simulink model "MMNNsExample2"  (R2014a)
settings: Solver=ode45  SolverMode=SingleTasking  StartTime=0.0  StopTime=5  RelTol=1e-5
(part 1 of 2)
settings Model: Creator=Administrator  LastModifiedBy=Administrator
settings SolverCC: ZeroCrossControl=DisableAll
settings OptimizationCC: BlockReduction=off  BooleanDataType=off
settings DebuggingCC: SaveWithParameterizedLinksMsg=none  UnderspecifiedInitializationDetection=Classic  SignalResolutionControl=TryResolveAllWithWarning  MaxConsecutiveZCsMsg=none  SolverPrmCheckMsg=none
settings HardwareCC: TargetUnknown=on

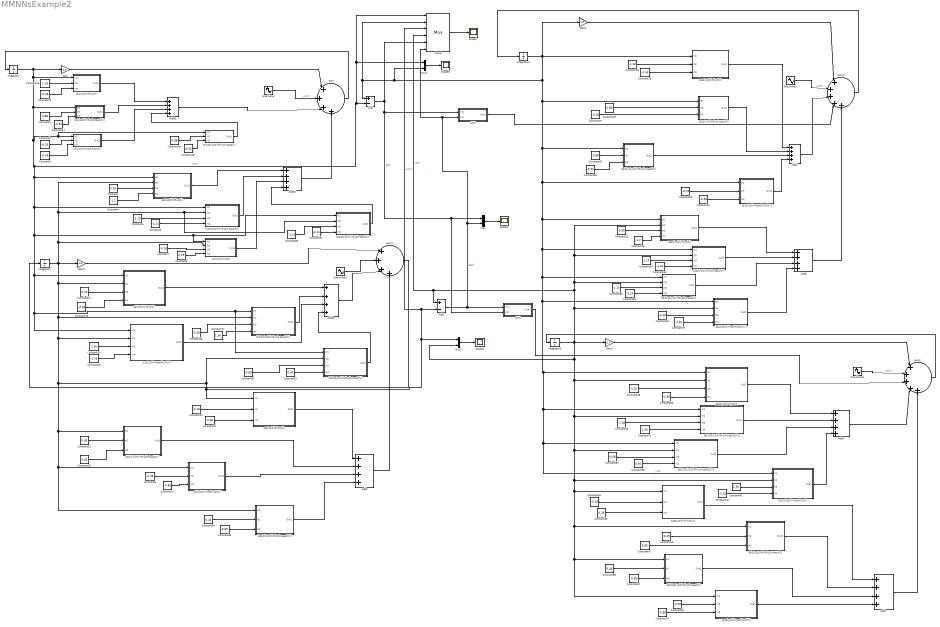
== system MMNNsExample2 ==
  22c21(y2(t))*inst(f(y1(t)) : Subsystem
  2a11(y1(t))*f(y1(t)) : Subsystem
  2a12(y1(t))*f(y2(t)) : Subsystem
  2a21(y2(t))*y1(t)1 : Subsystem
  2a22(x2(t))*f(x2(t))1 : Subsystem
  2b(1)11(y1(t))*f(y1(t-tau2(t))) : Subsystem
  2b(1)21(y2(t))*f(y1(t-tau1(t)))1 : Subsystem
  2b(1)22(y2(t))*f(y2(t-tau(t))1 : Subsystem
  2b(2)12(y1(t))*f(y2(t-tau2(t))) : Subsystem
  2b(2)21(y2(t))*f(y1(t-tau2(t)))1 : Subsystem
  2b(2)22(y2(t))*f(y2(t-tau2(t)) : Subsystem
  2b11(y1(t))*f(y1(t-tau(t))) : Subsystem
  2b12(y1(t))*f(y2(t-tau1(t))) : Subsystem
  2c11(y1(t))*inst(f(y1(t)))1 : Subsystem
  2c12(y1(t))*inst(f(y2(t))))1 : Subsystem
  2c22(y2(t))*inst(f(y2(t))) : Subsystem
  Add : Sum  Inputs=+-
  Add01 : Sum  Inputs=++++
      settings: AttributesFormatString=%<Name>
  Add02 : Sum  Inputs=++++
      settings: AttributesFormatString=%<Name>
  Add03 : Sum  Inputs=++++
      settings: AttributesFormatString=%<Name>
  Add1 : Sum  Inputs=+-
  Add{3..7} (5 alike) : Sum  Inputs=++++
      settings: AttributesFormatString=%<Name>
  Constant : Constant  Value=0.95
  Constant{1,26,48,62} (4 alike) : Constant  Value=0.88
  Constant{10,15,24,39} (4 alike) : Constant  Value=-0.85
      Constant15 settings: AttributesFormatString=%<Name>
      Constant39 settings: AttributesFormatString=%<Name>
  Constant11 : Constant  Value=0.25
      settings: AttributesFormatString=%<Name>
  Constant12 : Constant  Value=1.18
  Constant13 : Constant  Value=-0.45
  Constant{14,27,49,63} (4 alike) : Constant  Value=-0.92
  Constant16 : Constant  Value=-1.68
  Constant17 : Constant  Value=1.56
  Constant18 : Constant  Value=2.56
  Constant19 : Constant  Value=-1.76
  Constant2 : Constant  Value=-0.25
  Constant{7,20,36,44} (4 alike) : Constant  Value=-0.18
  Constant21 : Constant  Value=0.36
  Constant{22,46,54,56} (4 alike) : Constant  Value=0.45
  Constant{23,47,55,57} (4 alike) : Constant  Value=0.85
  Constant25 : Constant  Value=-0.35
  Constant28 : Constant  Value=1.18
  Constant29 : Constant  Value=-0.45
  Constant3 : Constant  Value=-0.56
  Constant30 : Constant  Value=-0.25
  Constant31 : Constant  Value=-0.56
  Constant32 : Constant  Value=0.95
  Constant33 : Constant  Value=-1.2
  Constant34 : Constant  Value=1.15
  Constant35 : Constant  Value=-1.24
  Constant37 : Constant  Value=0.15
  Constant38 : Constant  Value=0.25
      settings: AttributesFormatString=%<Name>
  Constant4 : Constant  Value=-1.2
  Constant40 : Constant  Value=-1.68
  Constant41 : Constant  Value=1.56
  Constant42 : Constant  Value=2.56
  Constant43 : Constant  Value=-1.76
  Constant45 : Constant  Value=0.36
  Constant5 : Constant  Value=1.15
  Constant50 : Constant  Value=-1.15
  Constant51 : Constant  Value=-2.24
  Constant52 : Constant  Value=-0.68
  Constant53 : Constant  Value=0.56
  Constant58 : Constant  Value=0.56
  Constant59 : Constant  Value=-0.68
  Constant6 : Constant  Value=-1.24
  Constant60 : Constant  Value=-1.15
  Constant61 : Constant  Value=-2.24
  Constant8 : Constant  Value=0.15
  Constant9 : Constant  Value=-0.35
  Gain : Gain  Gain=-4.5
  Gain1 : Gain  Gain=-2.5
      settings: AttributesFormatString=|
      | %<Name>
      | %<Gain>
  Gain2 : Gain  Gain=-4.5
      settings: AttributesFormatString=%<Gain>
  Gain3 : Gain  Gain=-2.5
      settings: AttributesFormatString=|
      | %<Name>
      | %<Gain>
  Integrator : Integrator  InitialCondition=0.4
      settings: AttributesFormatString=|
      | %<Name>
      | %<InitialCondition>
  Integrator1 : Integrator  InitialCondition=0.6
      settings: AttributesFormatString=|
      | %<Name>
      | %<InitialCondition>
  Integrator2 : Integrator  InitialCondition=5
      settings: AttributesFormatString=|
      | %<Name>
      | %<InitialCondition>
  Integrator3 : Integrator  InitialCondition=2
      settings: AttributesFormatString=|
      | %<Name>
      | %<InitialCondition>
  Mux : Mux  Inputs=2
  Mux1 : Mux  Inputs=2
  Mux2 : Mux  Inputs=2
  Mux3 : Mux  Inputs=6
  Scope{1..4} (4 alike) : Scope
      Scope1 settings: MaxDataPoints=50000000
      Scope2 settings: AttributesFormatString=%<Name>  YMin=-0.5  MaxDataPoints=50000000
      Scope3 settings: MaxDataPoints=50000000
      Scope4 settings: AttributesFormatString=%<Name>  YMin=-1  SaveName=ScopeData2  MaxDataPoints=50000000
  Sine Wave : Sin  SampleTime=0
      settings: AttributesFormatString=%<Name>
  Sine Wave1 : Sin  Phase=1  SampleTime=0.5*pi
      settings: AttributesFormatString=%<Name>
  Sine Wave2 : Sin  SampleTime=0
  Sine Wave3 : Sin  Phase=pi/2  SampleTime=0
  Sum : Sum  Inputs=|++++
      settings: AttributesFormatString=%<Name>
  Sum1 : Sum  Inputs=|++++
      settings: AttributesFormatString=%<Name>
  Sum2 : Sum  Inputs=|+++++
      settings: AttributesFormatString=%<Name>
  Sum3 : Sum  Inputs=|+++++
      settings: AttributesFormatString=%<Name>
  a11(x1(t))*f(x1(t)) : Subsystem
  a12(x1(t))*f(x2(t)) : Subsystem
  a21(x2(t))*f(x1(t)) : Subsystem
  a22(x2(t))*f(x2(t)) : Subsystem
  b(1)12(x1(t))*f(x2(t-tau1(t))) : Subsystem
  b(1)21(x2(t))*f(x1(t-tau1(t))) : Subsystem
  b(2)11(x1(t))*f(x1(t-tau2t))) : Subsystem
  b(2)12(x1(t))*f(x2(t-tau2(t))) : Subsystem
  b(2)21(x2(t))*f(x1(t-tau2(t))) : Subsystem
  b11(x1(t))*f(x1(t-tau1(t))) : Subsystem
  b22(1)(x2(t))*f(x2(t-tau1(t))) : Subsystem
  b22(2)(x2(t))*f(x2(t-tau2(t))) : Subsystem
  c11(x1(t))*inst(f(x1(t))) : Subsystem
  c12(x1(t))*x2(t) : Subsystem
  c21(x2(t))*inst(f(x1(t))) : Subsystem
  c22(x2(t))*inst(f(x2(t))) : Subsystem
  u1(t) : Subsystem
  u2(t) : Subsystem
  wires:
  a21(x2(t))*f(x1(t))/1(Out1) -> Add03/1
  Integrator/1 -> b(2)11(x1(t))*f(x1(t-tau2t)))/1(In1), c11(x1(t))*inst(f(x1(t)))/1(In1), a12(x1(t))*f(x2(t))/1(In1), b(1)12(x1(t))*f(x2(t-tau1(t)))/1(In1), c21(x2(t))*inst(f(x1(t)))/1(In1), b(2)21(x2(t))*f(x1(t-tau2(t)))/1(In1), b(1)21(x2(t))*f(x1(t-tau1(t)))/1(In1), a21(x2(t))*f(x1(t))/1(In1), b(2)12(x1(t))*f(x2(t-tau2(t)))/1(In1), c12(x1(t))*x2(t)/1(In1), Mux1/1, Mux3/1, Add/2, b11(x1(t))*f(x1(t-tau1(t)))/1(In1), a11(x1(t))*f(x1(t))/1(In1), Gain/1  "x1(t)"
  a12(x1(t))*f(x2(t))/1(Out1) -> Add02/1
  Add02/1 -> Sum/4
  Sine Wave/1 -> Sum/2  "sin(t)"
  Add01/1 -> Sum/3
  Sum/1 -> Integrator/1
  Gain/1 -> Sum/1
  Integrator1/1 -> b(2)12(x1(t))*f(x2(t-tau2(t)))/2(In2), b(1)12(x1(t))*f(x2(t-tau1(t)))/2(In2), a12(x1(t))*f(x2(t))/2(In2), c12(x1(t))*x2(t)/2(In2), Mux2/1, Mux3/3, Add1/2, a22(x2(t))*f(x2(t))/1(In1), b(2)21(x2(t))*f(x1(t-tau2(t)))/2(In2), b22(2)(x2(t))*f(x2(t-tau2(t)))/1(In1), c22(x2(t))*inst(f(x2(t)))/1(In1), b22(1)(x2(t))*f(x2(t-tau1(t)))/1(In1), c21(x2(t))*inst(f(x1(t)))/2(In2), b(1)21(x2(t))*f(x1(t-tau1(t)))/2(In2), a21(x2(t))*f(x1(t))/2(In2), Gain1/1  "x2(t)"
  Gain1/1 -> Sum1/1
  Sine Wave1/1 -> Sum1/2
  Add03/1 -> Sum1/3
  Add3/1 -> Sum1/4
  Gain2/1 -> Sum2/1
  Sum2/1 -> Integrator2/1
  Sine Wave3/1 -> Sum3/2  "cos(t)"
  Gain3/1 -> Sum3/1
  Integrator2/1 -> 2b(1)11(y1(t))*f(y1(t-tau2(t)))/1(In1), 2b(2)12(y1(t))*f(y2(t-tau2(t)))/1(In1), 2a21(y2(t))*y1(t)1/1(In1), 22c21(y2(t))*inst(f(y1(t))/1(In1), 2b(2)21(y2(t))*f(y1(t-tau2(t)))1/1(In1), 2b(1)21(y2(t))*f(y1(t-tau1(t)))1/1(In1), 2c12(y1(t))*inst(f(y2(t))))1/1(In1), 2b12(y1(t))*f(y2(t-tau1(t)))/1(In1), 2a12(y1(t))*f(y2(t))/1(In1), 2c11(y1(t))*inst(f(y1(t)))1/1(In1), 2b11(y1(t))*f(y1(t-tau(t)))/1(In1), Mux1/2, Add/1, Mux3/2, 2a11(y1(t))*f(y1(t))/1(In1), Gain2/1  "y1(t)"
  Sum3/1 -> Integrator3/1
  Add6/1 -> Sum3/4
  Add5/1 -> Sum2/5
  a11(x1(t))*f(x1(t))/1(Out1) -> Add01/1
  b11(x1(t))*f(x1(t-tau1(t)))/1(Out1) -> Add01/2
  c11(x1(t))*inst(f(x1(t)))/1(Out1) -> Add01/3
  b(1)12(x1(t))*f(x2(t-tau1(t)))/1(Out1) -> Add02/2
  c12(x1(t))*x2(t)/1(Out1) -> Add02/3
  2c12(y1(t))*inst(f(y2(t))))1/1(Out1) -> Add5/4
  b(1)21(x2(t))*f(x1(t-tau1(t)))/1(Out1) -> Add03/2
  c21(x2(t))*inst(f(x1(t)))/1(Out1) -> Add03/3
  b22(1)(x2(t))*f(x2(t-tau1(t)))/1(Out1) -> Add3/2
  c22(x2(t))*inst(f(x2(t)))/1(Out1) -> Add3/3
  a22(x2(t))*f(x2(t))/1(Out1) -> Add3/1
  2b(1)22(y2(t))*f(y2(t-tau(t))1/1(Out1) -> Add7/2
  Sine Wave2/1 -> Sum2/2  "sin(t)"
  Add4/1 -> Sum2/3
  Add/1 -> u1(t)/1(In1), u2(t)/2(In2), Mux/1, Mux3/5  "e1(t)"
  Add1/1 -> u2(t)/1(In1), Mux/2, u1(t)/2(In2), Mux3/6  "e2(t)"
  Sum1/1 -> Integrator1/1
  Mux/1 -> Scope2/1
  Add7/1 -> Sum3/5
  Constant12/1 -> a11(x1(t))*f(x1(t))/2(In2)
  Constant13/1 -> a11(x1(t))*f(x1(t))/3(In3)
  Constant1/1 -> b11(x1(t))*f(x1(t-tau1(t)))/2(In2)
  Constant14/1 -> b11(x1(t))*f(x1(t-tau1(t)))/3(In3)
  Constant2/1 -> c11(x1(t))*inst(f(x1(t)))/2(In2)
  Constant3/1 -> c11(x1(t))*inst(f(x1(t)))/3(In3)
  Constant/1 -> a12(x1(t))*f(x2(t))/3(In3)
  Constant4/1 -> a12(x1(t))*f(x2(t))/4(In4)
  Constant5/1 -> b(1)12(x1(t))*f(x2(t-tau1(t)))/3(In3)
  Constant6/1 -> b(1)12(x1(t))*f(x2(t-tau1(t)))/4(In4)
  Constant7/1 -> c12(x1(t))*x2(t)/3(In3)
  Constant8/1 -> c12(x1(t))*x2(t)/4(In4)
  Constant9/1 -> c22(x2(t))*inst(f(x2(t)))/2(In2)
  Constant10/1 -> c22(x2(t))*inst(f(x2(t)))/3(In3)
  Constant15/1 -> a21(x2(t))*f(x1(t))/4(In4)
  Constant11/1 -> a21(x2(t))*f(x1(t))/3(In3)
  Constant16/1 -> b(1)21(x2(t))*f(x1(t-tau1(t)))/3(In3)
  Constant17/1 -> b(1)21(x2(t))*f(x1(t-tau1(t)))/4(In4)
  Constant18/1 -> c21(x2(t))*inst(f(x1(t)))/3(In3)
  Constant19/1 -> c21(x2(t))*inst(f(x1(t)))/4(In4)
  Constant20/1 -> a22(x2(t))*f(x2(t))/2(In2)
  Constant21/1 -> a22(x2(t))*f(x2(t))/3(In3)
  Constant22/1 -> b22(1)(x2(t))*f(x2(t-tau1(t)))/2(In2)
  Constant23/1 -> b22(1)(x2(t))*f(x2(t-tau1(t)))/3(In3)
  Constant25/1 -> 2c22(y2(t))*inst(f(y2(t)))/2(In2)
  Constant24/1 -> 2c22(y2(t))*inst(f(y2(t)))/3(In3)
  2c22(y2(t))*inst(f(y2(t)))/1(Out1) -> Add7/4
  Constant28/1 -> 2a11(y1(t))*f(y1(t))/2(In2)
  Constant29/1 -> 2a11(y1(t))*f(y1(t))/3(In3)
  Constant26/1 -> 2b11(y1(t))*f(y1(t-tau(t)))/2(In2)
  Constant27/1 -> 2b11(y1(t))*f(y1(t-tau(t)))/3(In3)
  Constant31/1 -> 2c11(y1(t))*inst(f(y1(t)))1/3(In3)
  Constant30/1 -> 2c11(y1(t))*inst(f(y1(t)))1/2(In2)
  2a11(y1(t))*f(y1(t))/1(Out1) -> Add4/1
  2b11(y1(t))*f(y1(t-tau(t)))/1(Out1) -> Add4/2
  2c11(y1(t))*inst(f(y1(t)))1/1(Out1) -> Add4/4
  Constant32/1 -> 2a12(y1(t))*f(y2(t))/3(In3)
  Constant33/1 -> 2a12(y1(t))*f(y2(t))/4(In4)
  2a12(y1(t))*f(y2(t))/1(Out1) -> Add5/1
  Constant34/1 -> 2b12(y1(t))*f(y2(t-tau1(t)))/3(In3)
  Constant35/1 -> 2b12(y1(t))*f(y2(t-tau1(t)))/4(In4)
  2b12(y1(t))*f(y2(t-tau1(t)))/1(Out1) -> Add5/2
  Constant36/1 -> 2c12(y1(t))*inst(f(y2(t))))1/3(In3)
  Constant37/1 -> 2c12(y1(t))*inst(f(y2(t))))1/4(In4)
  Constant38/1 -> 2a21(y2(t))*y1(t)1/3(In3)
  Constant39/1 -> 2a21(y2(t))*y1(t)1/4(In4)
  Constant40/1 -> 2b(1)21(y2(t))*f(y1(t-tau1(t)))1/3(In3)
  Constant41/1 -> 2b(1)21(y2(t))*f(y1(t-tau1(t)))1/4(In4)
  2b(1)21(y2(t))*f(y1(t-tau1(t)))1/1(Out1) -> Add6/2
  Constant43/1 -> 22c21(y2(t))*inst(f(y1(t))/4(In4)
  Constant42/1 -> 22c21(y2(t))*inst(f(y1(t))/3(In3)
  22c21(y2(t))*inst(f(y1(t))/1(Out1) -> Add6/4
  2a21(y2(t))*y1(t)1/1(Out1) -> Add6/1
  Constant44/1 -> 2a22(x2(t))*f(x2(t))1/2(In2)
  Constant45/1 -> 2a22(x2(t))*f(x2(t))1/3(In3)
  2a22(x2(t))*f(x2(t))1/1(Out1) -> Add7/1
  Constant46/1 -> 2b(1)22(y2(t))*f(y2(t-tau(t))1/2(In2)
  Constant47/1 -> 2b(1)22(y2(t))*f(y2(t-tau(t))1/3(In3)
  Mux1/1 -> Scope3/1
  Mux2/1 -> Scope4/1
  u1(t)/1(Out1) -> Sum2/4
  Constant48/1 -> b(2)11(x1(t))*f(x1(t-tau2t)))/2(In2)
  Constant49/1 -> b(2)11(x1(t))*f(x1(t-tau2t)))/3(In3)
  b(2)11(x1(t))*f(x1(t-tau2t)))/1(Out1) -> Add01/4
  Constant51/1 -> b(2)12(x1(t))*f(x2(t-tau2(t)))/4(In4)
  Constant50/1 -> b(2)12(x1(t))*f(x2(t-tau2(t)))/3(In3)
  b(2)12(x1(t))*f(x2(t-tau2(t)))/1(Out1) -> Add02/4
  Constant53/1 -> b(2)21(x2(t))*f(x1(t-tau2(t)))/4(In4)
  Constant52/1 -> b(2)21(x2(t))*f(x1(t-tau2(t)))/3(In3)
  b(2)21(x2(t))*f(x1(t-tau2(t)))/1(Out1) -> Add03/4
  Constant55/1 -> b22(2)(x2(t))*f(x2(t-tau2(t)))/3(In3)
  Constant54/1 -> b22(2)(x2(t))*f(x2(t-tau2(t)))/2(In2)
  b22(2)(x2(t))*f(x2(t-tau2(t)))/1(Out1) -> Add3/4
  Constant57/1 -> 2b(2)22(y2(t))*f(y2(t-tau2(t))/3(In3)
  Integrator3/1 -> 2a12(y1(t))*f(y2(t))/2(In2), 2b12(y1(t))*f(y2(t-tau1(t)))/2(In2), 2b(2)12(y1(t))*f(y2(t-tau2(t)))/2(In2), Mux3/4, Add1/1, 2c12(y1(t))*inst(f(y2(t))))1/2(In2), Gain3/1, Mux2/2, 2a21(y2(t))*y1(t)1/2(In2), 2b(1)21(y2(t))*f(y1(t-tau1(t)))1/2(In2), 2b(2)21(y2(t))*f(y1(t-tau2(t)))1/2(In2), 2a22(x2(t))*f(x2(t))1/1(In1), 2c22(y2(t))*inst(f(y2(t)))/1(In1), 2b(2)22(y2(t))*f(y2(t-tau2(t))/1(In1), 2b(1)22(y2(t))*f(y2(t-tau(t))1/1(In1), 22c21(y2(t))*inst(f(y1(t))/2(In2)  "y2(t)"
  Constant56/1 -> 2b(2)22(y2(t))*f(y2(t-tau2(t))/2(In2)
  2b(2)22(y2(t))*f(y2(t-tau2(t))/1(Out1) -> Add7/3
  Constant59/1 -> 2b(2)21(y2(t))*f(y1(t-tau2(t)))1/3(In3)
  Constant58/1 -> 2b(2)21(y2(t))*f(y1(t-tau2(t)))1/4(In4)
  2b(2)21(y2(t))*f(y1(t-tau2(t)))1/1(Out1) -> Add6/3
  Constant61/1 -> 2b(2)12(y1(t))*f(y2(t-tau2(t)))/4(In4)
  Constant60/1 -> 2b(2)12(y1(t))*f(y2(t-tau2(t)))/3(In3)
  2b(2)12(y1(t))*f(y2(t-tau2(t)))/1(Out1) -> Add5/3
  Constant63/1 -> 2b(1)11(y1(t))*f(y1(t-tau2(t)))/3(In3)
  Constant62/1 -> 2b(1)11(y1(t))*f(y1(t-tau2(t)))/2(In2)
  2b(1)11(y1(t))*f(y1(t-tau2(t)))/1(Out1) -> Add4/3
  u2(t)/1(Out1) -> Sum3/3
  Mux3/1 -> Scope1/1

== system MMNNsExample2/22c21(y2(t))*inst(f(y1(t)) ==
  In1 : Inport
      settings: AttributesFormatString=%<Name>
  In2 : Inport  Port=2
      settings: AttributesFormatString=%<Name>
  In3 : Inport  Port=3
      settings: AttributesFormatString=%<Name>
  In4 : Inport  Port=4
      settings: AttributesFormatString=%<Name>
  Abs : Abs
  Subsystem : Subsystem
  Switch : Switch  Criteria=u2 > Threshold  Threshold=1
  Out1 : Outport
  wires:
  In1/1 -> Subsystem/2(In2)  "x1(t)"
  Subsystem/1(Out1) -> Out1/1
  Abs/1 -> Switch/2
  In3/1 -> Switch/1
  In4/1 -> Switch/3
  Switch/1 -> Subsystem/1(In1)
  In2/1 -> Abs/1  "x2(t)"

== system MMNNsExample2/2a11(y1(t))*f(y1(t)) ==
  In1 : Inport
  In2 : Inport  Port=2
  In3 : Inport  Port=3
  Abs3 : Abs
  Switch4 : Switch  Criteria=u2 > Threshold  Threshold=1
  a11(x1(t))*x1(t) : Subsystem
  Out1 : Outport
  wires:
  a11(x1(t))*x1(t)/1(Out1) -> Out1/1
  Abs3/1 -> Switch4/2
  In2/1 -> Switch4/1
  In3/1 -> Switch4/3
  In1/1 -> a11(x1(t))*x1(t)/2(In2), Abs3/1  "x1(t)"
  Switch4/1 -> a11(x1(t))*x1(t)/1(ln1)

== system MMNNsExample2/2a12(y1(t))*f(y2(t)) ==
  In1 : Inport
      settings: AttributesFormatString=%<Name>
  In2 : Inport  Port=2
      settings: AttributesFormatString=%<Name>
  In3 : Inport  Port=3
      settings: AttributesFormatString=%<Name>
  In4 : Inport  Port=4
      settings: AttributesFormatString=%<Name>
  Abs : Abs
  Subsystem : Subsystem
  Switch : Switch  Criteria=u2 > Threshold  Threshold=1
  Out1 : Outport
  wires:
  In1/1 -> Abs/1  "x1(t)"
  Switch/1 -> Subsystem/1(In1)
  In2/1 -> Subsystem/2(In2)  "x2(t)"
  Subsystem/1(Out1) -> Out1/1
  Abs/1 -> Switch/2
  In3/1 -> Switch/1
  In4/1 -> Switch/3

== system MMNNsExample2/2a21(y2(t))*y1(t)1 ==
  In1 : Inport
      settings: AttributesFormatString=%<Name>
  In2 : Inport  Port=2
      settings: AttributesFormatString=%<Name>
  In3 : Inport  Port=3
      settings: AttributesFormatString=%<Name>
  In4 : Inport  Port=4
      settings: AttributesFormatString=%<Name>
  Abs : Abs
      settings: AttributesFormatString=%<Name>
  Product : Product
      settings: AttributesFormatString=%<Name>
  Switch : Switch  Criteria=u2 > Threshold  Threshold=1
  f1(x1(t))=(|x+1|-|x-1|)/2 : Subsystem
  Out1 : Outport
      settings: AttributesFormatString=%<Name>
  wires:
  Product/1 -> Out1/1
  In2/1 -> Abs/1  "x2(t)"
  f1(x1(t))=(|x+1|-|x-1|)/2/1(Out1) -> Product/2
  In1/1 -> f1(x1(t))=(|x+1|-|x-1|)/2/1(In1)  "x1(t)"
  In4/1 -> Switch/1
  Switch/1 -> Product/1
  Abs/1 -> Switch/2
  In3/1 -> Switch/3

== system MMNNsExample2/2a22(x2(t))*f(x2(t))1 ==
  In1 : Inport
  In2 : Inport  Port=2
  In3 : Inport  Port=3
  Abs3 : Abs
  Switch4 : Switch  Criteria=u2 > Threshold  Threshold=1
  a22(x2(t))*x2(t) : Subsystem
  Out1 : Outport
  wires:
  a22(x2(t))*x2(t)/1(Out1) -> Out1/1
  In1/1 -> a22(x2(t))*x2(t)/2(In2), Abs3/1  "x2(t)"
  Switch4/1 -> a22(x2(t))*x2(t)/1(ln1)
  Abs3/1 -> Switch4/2
  In3/1 -> Switch4/3
  In2/1 -> Switch4/1

== system MMNNsExample2/2b(1)11(y1(t))*f(y1(t-tau2(t))) ==
  In1 : Inport
  In2 : Inport  Port=2
  In3 : Inport  Port=3
  Abs1 : Abs
  Switch1 : Switch  Criteria=u2 > Threshold  Threshold=1
  x1(t)*b11(x1(t)) : Subsystem
  Out1 : Outport
  wires:
  In1/1 -> x1(t)*b11(x1(t))/2(In2), Abs1/1  "x1(t)"
  x1(t)*b11(x1(t))/1(Out1) -> Out1/1
  Switch1/1 -> x1(t)*b11(x1(t))/1(In1)  "b11(x1(t))"
  In3/1 -> Switch1/1
  In2/1 -> Switch1/3
  Abs1/1 -> Switch1/2

== system MMNNsExample2/2b(1)21(y2(t))*f(y1(t-tau1(t)))1 ==
  In1 : Inport
      settings: AttributesFormatString=%<Name>
  In2 : Inport  Port=2
      settings: AttributesFormatString=%<Name>
  In3 : Inport  Port=3
      settings: AttributesFormatString=%<Name>
  In4 : Inport  Port=4
      settings: AttributesFormatString=%<Name>
  Abs : Abs
  Subsystem : Subsystem
  Switch : Switch  Criteria=u2 > Threshold  Threshold=1
      settings: AttributesFormatString=%<Name>
  Out1 : Outport
  wires:
  In1/1 -> Subsystem/2(In2)  "x1(t)"
  In2/1 -> Abs/1  "x2(t)"
  Subsystem/1(Out1) -> Out1/1
  In4/1 -> Switch/3
  In3/1 -> Switch/1
  Abs/1 -> Switch/2
  Switch/1 -> Subsystem/1(In1)  "b21"

== system MMNNsExample2/2b(1)22(y2(t))*f(y2(t-tau(t))1 ==
  In1 : Inport
  In2 : Inport  Port=2
  In3 : Inport  Port=3
  Abs1 : Abs
  Switch1 : Switch  Criteria=u2 > Threshold  Threshold=1
  x2(t)*b22(x2(t)) : Subsystem
  Out1 : Outport
  wires:
  In1/1 -> Abs1/1, x2(t)*b22(x2(t))/2(In2)  "x2(t)"
  x2(t)*b22(x2(t))/1(Out1) -> Out1/1
  In2/1 -> Switch1/1
  Abs1/1 -> Switch1/2
  In3/1 -> Switch1/3
  Switch1/1 -> x2(t)*b22(x2(t))/1(In1)

== system MMNNsExample2/2b(2)12(y1(t))*f(y2(t-tau2(t))) ==
  In1 : Inport
  In2 : Inport  Port=2
  In3 : Inport  Port=3
  In4 : Inport  Port=4
  Abs : Abs
  Subsystem : Subsystem
  Switch : Switch  Criteria=u2 > Threshold  Threshold=1
  Out1 : Outport
      settings: AttributesFormatString=%<Name>
  wires:
  Subsystem/1(Out1) -> Out1/1
  In3/1 -> Switch/1
  In4/1 -> Switch/3
  Switch/1 -> Subsystem/1(In1)  "b12"
  Abs/1 -> Switch/2
  In1/1 -> Abs/1  "x1(t)"
  In2/1 -> Subsystem/2(In2)

== system MMNNsExample2/2b(2)21(y2(t))*f(y1(t-tau2(t)))1 ==
  In1 : Inport
      settings: AttributesFormatString=%<Name>
  In2 : Inport  Port=2
      settings: AttributesFormatString=%<Name>
  In3 : Inport  Port=3
      settings: AttributesFormatString=%<Name>
  In4 : Inport  Port=4
      settings: AttributesFormatString=%<Name>
  Abs : Abs
  Subsystem : Subsystem
  Switch : Switch  Criteria=u2 > Threshold  Threshold=1
      settings: AttributesFormatString=%<Name>
  Out1 : Outport
  wires:
  In1/1 -> Subsystem/2(In2)  "x1(t)"
  In2/1 -> Abs/1  "x2(t)"
  Subsystem/1(Out1) -> Out1/1
  In4/1 -> Switch/3
  In3/1 -> Switch/1
  Abs/1 -> Switch/2
  Switch/1 -> Subsystem/1(In1)  "b21"

== system MMNNsExample2/2b(2)22(y2(t))*f(y2(t-tau2(t)) ==
  In1 : Inport
  In2 : Inport  Port=2
  In3 : Inport  Port=3
  Abs1 : Abs
  Switch1 : Switch  Criteria=u2 > Threshold  Threshold=1
  x2(t)*b22(x2(t)) : Subsystem
  Out1 : Outport
  wires:
  In1/1 -> Abs1/1, x2(t)*b22(x2(t))/2(In2)  "x2(t)"
  x2(t)*b22(x2(t))/1(Out1) -> Out1/1
  In2/1 -> Switch1/1
  Abs1/1 -> Switch1/2
  In3/1 -> Switch1/3
  Switch1/1 -> x2(t)*b22(x2(t))/1(In1)

== system MMNNsExample2/2b11(y1(t))*f(y1(t-tau(t))) ==
  In1 : Inport
  In2 : Inport  Port=2
  In3 : Inport  Port=3
  Abs1 : Abs
  Switch1 : Switch  Criteria=u2 > Threshold  Threshold=1
  x1(t)*b11(x1(t)) : Subsystem
  Out1 : Outport
  wires:
  In1/1 -> x1(t)*b11(x1(t))/2(In2), Abs1/1  "x1(t)"
  x1(t)*b11(x1(t))/1(Out1) -> Out1/1
  Switch1/1 -> x1(t)*b11(x1(t))/1(In1)  "b11(x1(t))"
  In3/1 -> Switch1/1
  In2/1 -> Switch1/3
  Abs1/1 -> Switch1/2

== system MMNNsExample2/2b12(y1(t))*f(y2(t-tau1(t))) ==
  In1 : Inport
  In2 : Inport  Port=2
  In3 : Inport  Port=3
  In4 : Inport  Port=4
  Abs : Abs
  Subsystem : Subsystem
  Switch : Switch  Criteria=u2 > Threshold  Threshold=1
  Out1 : Outport
      settings: AttributesFormatString=%<Name>
  wires:
  Subsystem/1(Out1) -> Out1/1
  In3/1 -> Switch/1
  In4/1 -> Switch/3
  Switch/1 -> Subsystem/1(In1)  "b12"
  Abs/1 -> Switch/2
  In1/1 -> Abs/1  "x1(t)"
  In2/1 -> Subsystem/2(In2)

== system MMNNsExample2/2c11(y1(t))*inst(f(y1(t)))1 ==
  In1 : Inport
      settings: AttributesFormatString=%<Name>
  In2 : Inport  Port=2
      settings: AttributesFormatString=%<Name>
  In3 : Inport  Port=3
      settings: AttributesFormatString=%<Name>
  Abs3 : Abs
  Switch4 : Switch  Criteria=u2 > Threshold  Threshold=1
  c11*inst(f1(x1(t))) : Subsystem
  Out1 : Outport
  wires:
  c11*inst(f1(x1(t)))/1(Out1) -> Out1/1
  In1/1 -> Abs3/1, c11*inst(f1(x1(t)))/2(In2)  "x1(t)"
  Abs3/1 -> Switch4/2
  Switch4/1 -> c11*inst(f1(x1(t)))/1(In1)  "c11"
  In2/1 -> Switch4/1
  In3/1 -> Switch4/3

== system MMNNsExample2/2c12(y1(t))*inst(f(y2(t))))1 ==
  In1 : Inport
      settings: AttributesFormatString=%<Name>
  In2 : Inport  Port=2
      settings: AttributesFormatString=%<Name>
  In3 : Inport  Port=3
      settings: AttributesFormatString=%<Name>
  In4 : Inport  Port=4
      settings: AttributesFormatString=%<Name>
  Abs : Abs
  Subsystem : Subsystem
  Switch : Switch  Criteria=u2 > Threshold  Threshold=1
  Out1 : Outport
  wires:
  In1/1 -> Abs/1  "x1(t)"
  In2/1 -> Subsystem/2(In2)  "x2(t)"
  Subsystem/1(Out1) -> Out1/1
  Switch/1 -> Subsystem/1(In1)
  Abs/1 -> Switch/2
  In3/1 -> Switch/1
  In4/1 -> Switch/3

== system MMNNsExample2/2c22(y2(t))*inst(f(y2(t))) ==
  In1 : Inport
  In2 : Inport  Port=2
  In3 : Inport  Port=3
  Abs3 : Abs
  Switch4 : Switch  Criteria=u2 > Threshold  Threshold=1
  c22*inst(f2(x2(t))) : Subsystem
  Out1 : Outport
  wires:
  c22*inst(f2(x2(t)))/1(Out1) -> Out1/1
  In1/1 -> c22*inst(f2(x2(t)))/2(In2), Abs3/1  "x2(t)"
  Switch4/1 -> c22*inst(f2(x2(t)))/1(In1)  "c11"
  In2/1 -> Switch4/1
  Abs3/1 -> Switch4/2
  In3/1 -> Switch4/3

== system MMNNsExample2/a11(x1(t))*f(x1(t)) ==
  In1 : Inport
  In2 : Inport  Port=2
  In3 : Inport  Port=3
  Abs3 : Abs
  Switch4 : Switch  Criteria=u2 > Threshold  Threshold=1
  a11(x1(t))*x1(t) : Subsystem
  Out1 : Outport
  wires:
  a11(x1(t))*x1(t)/1(Out1) -> Out1/1
  Abs3/1 -> Switch4/2
  In2/1 -> Switch4/1
  In3/1 -> Switch4/3
  In1/1 -> a11(x1(t))*x1(t)/2(In2), Abs3/1  "x1(t)"
  Switch4/1 -> a11(x1(t))*x1(t)/1(ln1)

== system MMNNsExample2/a12(x1(t))*f(x2(t)) ==
  In1 : Inport
      settings: AttributesFormatString=%<Name>
  In2 : Inport  Port=2
      settings: AttributesFormatString=%<Name>
  In3 : Inport  Port=3
      settings: AttributesFormatString=%<Name>
  In4 : Inport  Port=4
      settings: AttributesFormatString=%<Name>
  Abs : Abs
  Subsystem : Subsystem
  Switch : Switch  Criteria=u2 > Threshold  Threshold=1
  Out1 : Outport
  wires:
  In1/1 -> Abs/1  "x1(t)"
  Switch/1 -> Subsystem/1(In1)
  In2/1 -> Subsystem/2(In2)  "x2(t)"
  Subsystem/1(Out1) -> Out1/1
  Abs/1 -> Switch/2
  In3/1 -> Switch/1
  In4/1 -> Switch/3

== system MMNNsExample2/a21(x2(t))*f(x1(t)) ==
  In1 : Inport
      settings: AttributesFormatString=%<Name>
  In2 : Inport  Port=2
      settings: AttributesFormatString=%<Name>
  In3 : Inport  Port=3
      settings: AttributesFormatString=%<Name>
  In4 : Inport  Port=4
      settings: AttributesFormatString=%<Name>
  Abs : Abs
      settings: AttributesFormatString=%<Name>
  Product : Product
      settings: AttributesFormatString=%<Name>
  Switch : Switch  Criteria=u2 > Threshold  Threshold=1
  f1(x1(t))=(|x+1|-|x-1|)/2 : Subsystem
  Out1 : Outport
      settings: AttributesFormatString=%<Name>
  wires:
  Product/1 -> Out1/1
  In2/1 -> Abs/1  "x2(t)"
  f1(x1(t))=(|x+1|-|x-1|)/2/1(Out1) -> Product/2
  In1/1 -> f1(x1(t))=(|x+1|-|x-1|)/2/1(In1)  "x1(t)"
  In4/1 -> Switch/1
  Switch/1 -> Product/1
  Abs/1 -> Switch/2
  In3/1 -> Switch/3

== system MMNNsExample2/a22(x2(t))*f(x2(t)) ==
  In1 : Inport
  In2 : Inport  Port=2
  In3 : Inport  Port=3
  Abs3 : Abs
  Switch4 : Switch  Criteria=u2 > Threshold  Threshold=1
  a22(x2(t))*x2(t) : Subsystem
  Out1 : Outport
  wires:
  a22(x2(t))*x2(t)/1(Out1) -> Out1/1
  In1/1 -> a22(x2(t))*x2(t)/2(In2), Abs3/1  "x2(t)"
  Switch4/1 -> a22(x2(t))*x2(t)/1(ln1)
  Abs3/1 -> Switch4/2
  In3/1 -> Switch4/3
  In2/1 -> Switch4/1

== system MMNNsExample2/b(1)12(x1(t))*f(x2(t-tau1(t))) ==
  In1 : Inport
  In2 : Inport  Port=2
  In3 : Inport  Port=3
  In4 : Inport  Port=4
  Abs : Abs
  Subsystem : Subsystem
  Switch : Switch  Criteria=u2 > Threshold  Threshold=1
  Out1 : Outport
      settings: AttributesFormatString=%<Name>
  wires:
  Subsystem/1(Out1) -> Out1/1
  In3/1 -> Switch/1
  In4/1 -> Switch/3
  Switch/1 -> Subsystem/1(In1)  "b12"
  Abs/1 -> Switch/2
  In1/1 -> Abs/1  "x1(t)"
  In2/1 -> Subsystem/2(In2)

== system MMNNsExample2/b(1)21(x2(t))*f(x1(t-tau1(t))) ==
  In1 : Inport
      settings: AttributesFormatString=%<Name>
  In2 : Inport  Port=2
      settings: AttributesFormatString=%<Name>
  In3 : Inport  Port=3
      settings: AttributesFormatString=%<Name>
  In4 : Inport  Port=4
      settings: AttributesFormatString=%<Name>
  Abs : Abs
  Subsystem : Subsystem
  Switch : Switch  Criteria=u2 > Threshold  Threshold=1
      settings: AttributesFormatString=%<Name>
  Out1 : Outport
  wires:
  In1/1 -> Subsystem/2(In2)  "x1(t)"
  In2/1 -> Abs/1  "x2(t)"
  Subsystem/1(Out1) -> Out1/1
  In4/1 -> Switch/3
  In3/1 -> Switch/1
  Abs/1 -> Switch/2
  Switch/1 -> Subsystem/1(In1)  "b21"

== system MMNNsExample2/b(2)11(x1(t))*f(x1(t-tau2t))) ==
  In1 : Inport
  In2 : Inport  Port=2
  In3 : Inport  Port=3
  Abs1 : Abs
  Switch1 : Switch  Criteria=u2 > Threshold  Threshold=1
  x1(t)*b11(x1(t)) : Subsystem
  Out1 : Outport
  wires:
  In1/1 -> x1(t)*b11(x1(t))/2(In2), Abs1/1  "x1(t)"
  x1(t)*b11(x1(t))/1(Out1) -> Out1/1
  Switch1/1 -> x1(t)*b11(x1(t))/1(In1)  "b11(x1(t))"
  In3/1 -> Switch1/1
  In2/1 -> Switch1/3
  Abs1/1 -> Switch1/2

== system MMNNsExample2/b(2)12(x1(t))*f(x2(t-tau2(t))) ==
  In1 : Inport
  In2 : Inport  Port=2
  In3 : Inport  Port=3
  In4 : Inport  Port=4
  Abs : Abs
  Subsystem : Subsystem
  Switch : Switch  Criteria=u2 > Threshold  Threshold=1
  Out1 : Outport
      settings: AttributesFormatString=%<Name>
  wires:
  Subsystem/1(Out1) -> Out1/1
  In3/1 -> Switch/1
  In4/1 -> Switch/3
  Switch/1 -> Subsystem/1(In1)  "b12"
  Abs/1 -> Switch/2
  In1/1 -> Abs/1  "x1(t)"
  In2/1 -> Subsystem/2(In2)

== system MMNNsExample2/b(2)21(x2(t))*f(x1(t-tau2(t))) ==
  In1 : Inport
      settings: AttributesFormatString=%<Name>
  In2 : Inport  Port=2
      settings: AttributesFormatString=%<Name>
  In3 : Inport  Port=3
      settings: AttributesFormatString=%<Name>
  In4 : Inport  Port=4
      settings: AttributesFormatString=%<Name>
  Abs : Abs
  Subsystem : Subsystem
  Switch : Switch  Criteria=u2 > Threshold  Threshold=1
      settings: AttributesFormatString=%<Name>
  Out1 : Outport
  wires:
  In1/1 -> Subsystem/2(In2)  "x1(t)"
  In2/1 -> Abs/1  "x2(t)"
  Subsystem/1(Out1) -> Out1/1
  In4/1 -> Switch/3
  In3/1 -> Switch/1
  Abs/1 -> Switch/2
  Switch/1 -> Subsystem/1(In1)  "b21"

== system MMNNsExample2/b11(x1(t))*f(x1(t-tau1(t))) ==
  In1 : Inport
  In2 : Inport  Port=2
  In3 : Inport  Port=3
  Abs1 : Abs
  Switch1 : Switch  Criteria=u2 > Threshold  Threshold=1
  x1(t)*b11(x1(t)) : Subsystem
  Out1 : Outport
  wires:
  In1/1 -> x1(t)*b11(x1(t))/2(In2), Abs1/1  "x1(t)"
  x1(t)*b11(x1(t))/1(Out1) -> Out1/1
  Switch1/1 -> x1(t)*b11(x1(t))/1(In1)  "b11(x1(t))"
  In3/1 -> Switch1/1
  In2/1 -> Switch1/3
  Abs1/1 -> Switch1/2

== system MMNNsExample2/b22(1)(x2(t))*f(x2(t-tau1(t))) ==
  In1 : Inport
  In2 : Inport  Port=2
  In3 : Inport  Port=3
  Abs1 : Abs
  Switch1 : Switch  Criteria=u2 > Threshold  Threshold=1
  x2(t)*b22(x2(t)) : Subsystem
  Out1 : Outport
  wires:
  In1/1 -> Abs1/1, x2(t)*b22(x2(t))/2(In2)  "x2(t)"
  x2(t)*b22(x2(t))/1(Out1) -> Out1/1
  In2/1 -> Switch1/1
  Abs1/1 -> Switch1/2
  In3/1 -> Switch1/3
  Switch1/1 -> x2(t)*b22(x2(t))/1(In1)

== system MMNNsExample2/b22(2)(x2(t))*f(x2(t-tau2(t))) ==
  In1 : Inport
  In2 : Inport  Port=2
  In3 : Inport  Port=3
  Abs1 : Abs
  Switch1 : Switch  Criteria=u2 > Threshold  Threshold=1
  x2(t)*b22(x2(t)) : Subsystem
  Out1 : Outport
  wires:
  In1/1 -> Abs1/1, x2(t)*b22(x2(t))/2(In2)  "x2(t)"
  x2(t)*b22(x2(t))/1(Out1) -> Out1/1
  In2/1 -> Switch1/1
  Abs1/1 -> Switch1/2
  In3/1 -> Switch1/3
  Switch1/1 -> x2(t)*b22(x2(t))/1(In1)

== system MMNNsExample2/c11(x1(t))*inst(f(x1(t))) ==
  In1 : Inport
      settings: AttributesFormatString=%<Name>
  In2 : Inport  Port=2
      settings: AttributesFormatString=%<Name>
  In3 : Inport  Port=3
      settings: AttributesFormatString=%<Name>
  Abs3 : Abs
  Switch4 : Switch  Criteria=u2 > Threshold  Threshold=1
  c11*inst(f1(x1(t))) : Subsystem
  Out1 : Outport
  wires:
  c11*inst(f1(x1(t)))/1(Out1) -> Out1/1
  In1/1 -> Abs3/1, c11*inst(f1(x1(t)))/2(In2)  "x1(t)"
  Abs3/1 -> Switch4/2
  Switch4/1 -> c11*inst(f1(x1(t)))/1(In1)  "c11"
  In2/1 -> Switch4/1
  In3/1 -> Switch4/3

== system MMNNsExample2/c12(x1(t))*x2(t) ==
  In1 : Inport
      settings: AttributesFormatString=%<Name>
  In2 : Inport  Port=2
      settings: AttributesFormatString=%<Name>
  In3 : Inport  Port=3
      settings: AttributesFormatString=%<Name>
  In4 : Inport  Port=4
      settings: AttributesFormatString=%<Name>
  Abs : Abs
  Subsystem : Subsystem
  Switch : Switch  Criteria=u2 > Threshold  Threshold=1
  Out1 : Outport
  wires:
  In1/1 -> Abs/1  "x1(t)"
  In2/1 -> Subsystem/2(In2)  "x2(t)"
  Subsystem/1(Out1) -> Out1/1
  Switch/1 -> Subsystem/1(In1)
  Abs/1 -> Switch/2
  In3/1 -> Switch/1
  In4/1 -> Switch/3

== system MMNNsExample2/c21(x2(t))*inst(f(x1(t))) ==
  In1 : Inport
      settings: AttributesFormatString=%<Name>
  In2 : Inport  Port=2
      settings: AttributesFormatString=%<Name>
  In3 : Inport  Port=3
      settings: AttributesFormatString=%<Name>
  In4 : Inport  Port=4
      settings: AttributesFormatString=%<Name>
  Abs : Abs
  Subsystem : Subsystem
  Switch : Switch  Criteria=u2 > Threshold  Threshold=1
  Out1 : Outport
  wires:
  In1/1 -> Subsystem/2(In2)  "x1(t)"
  Subsystem/1(Out1) -> Out1/1
  Abs/1 -> Switch/2
  In3/1 -> Switch/1
  In4/1 -> Switch/3
  Switch/1 -> Subsystem/1(In1)
  In2/1 -> Abs/1  "x2(t)"

== system MMNNsExample2/c22(x2(t))*inst(f(x2(t))) ==
  In1 : Inport
  In2 : Inport  Port=2
  In3 : Inport  Port=3
  Abs3 : Abs
  Switch4 : Switch  Criteria=u2 > Threshold  Threshold=1
  c22*inst(f2(x2(t))) : Subsystem
  Out1 : Outport
  wires:
  c22*inst(f2(x2(t)))/1(Out1) -> Out1/1
  In1/1 -> c22*inst(f2(x2(t)))/2(In2), Abs3/1  "x2(t)"
  Switch4/1 -> c22*inst(f2(x2(t)))/1(In1)  "c11"
  In2/1 -> Switch4/1
  Abs3/1 -> Switch4/2
  In3/1 -> Switch4/3

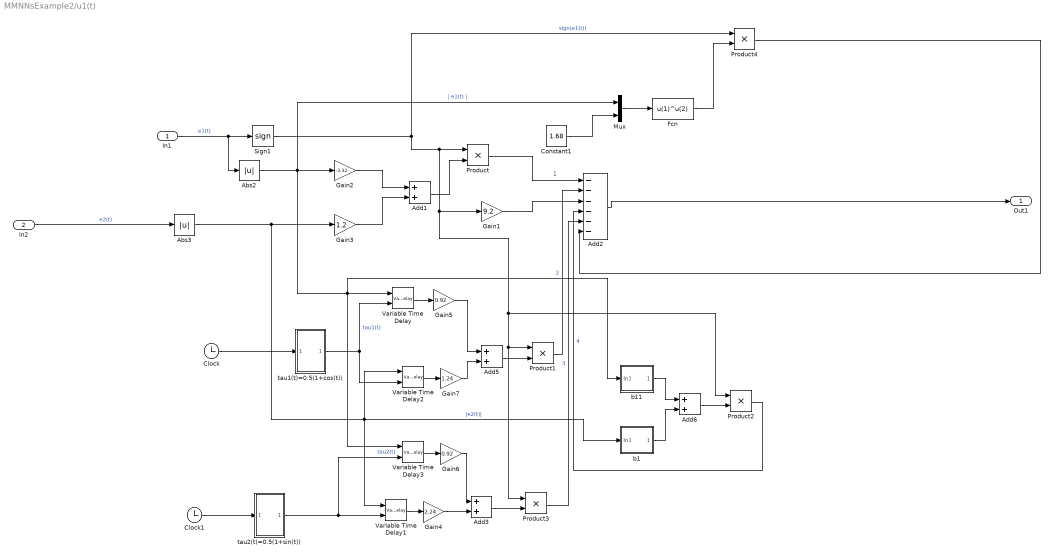
== system MMNNsExample2/u1(t) ==
  note: 1
  In1 : Inport
  In2 : Inport  Port=2
  Abs2 : Abs
  Abs3 : Abs
  Add{1,3,5..6} (4 alike) : Sum
  Add2 : Sum  Inputs=------
  Clock : Clock
  Clock1 : Clock
  Constant1 : Constant  Value=1.68
  Fcn : Fcn  Expr=u(1)^u(2)
  Gain1 : Gain  Gain=9.2
      settings: AttributesFormatString=%<Gain>
  Gain2 : Gain  Gain=-3.32
      settings: AttributesFormatString=%<Gain>
  Gain3 : Gain  Gain=1.2
      settings: AttributesFormatString=%<Gain>
  Gain4 : Gain  Gain=2.24
      settings: AttributesFormatString=%<Gain>
  Gain5 : Gain  Gain=0.92
      settings: AttributesFormatString=%<Gain>
  Gain6 : Gain  Gain=0.92
      settings: AttributesFormatString=%<Gain>
  Gain7 : Gain  Gain=1.24
      settings: AttributesFormatString=%<Gain>
  Mux : Mux  Inputs=2
  Product{,1..4} (5 alike) : Product
  Sign1 : Signum
  Variable Time Delay{,1..3} (4 alike) : VariableTransportDelay  MaximumDelay=10  MaximumPoints=2^20
  b1 : Subsystem
  b11 : Subsystem
  tau1(t)=0.5(1+cos(t)) : Subsystem
  tau2(t)=0.5(1+sin(t)) : Subsystem
  Out1 : Outport
  wires:
  In1/1 -> Abs2/1, Sign1/1  "e1(t)"
  Gain3/1 -> Add1/2
  Gain2/1 -> Add1/1
  Sign1/1 -> Gain1/1, Product2/1, Product3/1, Product1/1, Product/1, Product4/1  "sign(e1(t))"
  Add1/1 -> Product/2
  Product/1 -> Add2/1
  Abs2/1 -> Mux/1, Variable Time Delay/1, Variable Time Delay3/1, b11/1(In1), Gain2/1  "｜e1(t)｜"
  Variable Time Delay/1 -> Gain5/1
  Abs3/1 -> Variable Time Delay2/1, b1/1(In1), Variable Time Delay1/1, Gain3/1  "|e2(t)|"
  Gain5/1 -> Add5/1
  Gain7/1 -> Add5/2
  Add5/1 -> Product1/2
  Product1/1 -> Add2/2  "2"
  In2/1 -> Abs3/1  "e2(t)"
  b11/1(Out1) -> Add6/1
  b1/1(Out1) -> Add6/2
  Add6/1 -> Product2/2
  Product2/1 -> Add2/4  "4"
  Add2/1 -> Out1/1
  Clock1/1 -> tau2(t)=0.5(1+sin(t))/1(In1)
  tau2(t)=0.5(1+sin(t))/1(Out1) -> Variable Time Delay3/2, Variable Time Delay1/2  "tau2(t)"
  Clock/1 -> tau1(t)=0.5(1+cos(t))/1(In1)
  tau1(t)=0.5(1+cos(t))/1(Out1) -> Variable Time Delay/2, Variable Time Delay2/2  "tau1(t)"
  Product3/1 -> Add2/5  "3"
  Constant1/1 -> Mux/2
  Mux/1 -> Fcn/1
  Variable Time Delay2/1 -> Gain7/1
  Variable Time Delay1/1 -> Gain4/1
  Variable Time Delay3/1 -> Gain6/1
  Gain6/1 -> Add3/1
  Gain4/1 -> Add3/2
  Add3/1 -> Product3/2
  Gain1/1 -> Add2/3
  Fcn/1 -> Product4/2
  Product4/1 -> Add2/6

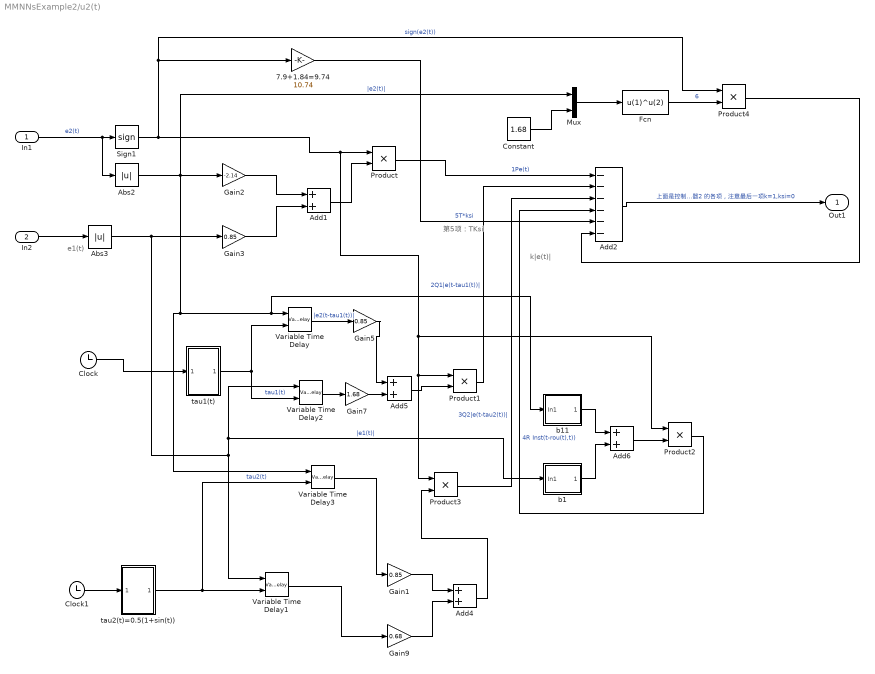
== system MMNNsExample2/u2(t) ==
  note: k|e(t)|
  note: 第5项：TKsi
  note: e1(t)
  In1 : Inport
  In2 : Inport  Port=2
  7.9+1.84=9.74 : Gain  Gain=10.74
      settings: AttributesFormatString=%<Gain>
  Abs2 : Abs
  Abs3 : Abs
  Add{1,4..6} (4 alike) : Sum
  Add2 : Sum  Inputs=------
  Clock : Clock
  Clock1 : Clock
  Constant : Constant  Value=1.68
  Fcn : Fcn  Expr=u(1)^u(2)
  Gain1 : Gain  Gain=0.85
      settings: AttributesFormatString=%<Gain>
  Gain2 : Gain  Gain=-2.14
      settings: AttributesFormatString=%<Gain>
  Gain3 : Gain  Gain=0.85
      settings: AttributesFormatString=%<Gain>
  Gain5 : Gain  Gain=0.85
      settings: AttributesFormatString=%<Gain>
  Gain7 : Gain  Gain=1.68
      settings: AttributesFormatString=%<Gain>
  Gain9 : Gain  Gain=0.68
      settings: AttributesFormatString=%<Gain>
  Mux : Mux  Inputs=2
  Product{,1..4} (5 alike) : Product
  Sign1 : Signum
  Variable Time Delay{,1..3} (4 alike) : VariableTransportDelay  MaximumDelay=10  MaximumPoints=2^20
  b1 : Subsystem
  b11 : Subsystem
  tau1(t) : Subsystem
  tau2(t)=0.5(1+sin(t)) : Subsystem
  Out1 : Outport
  wires:
  In1/1 -> Abs2/1, Sign1/1  "e2(t)"
  Gain3/1 -> Add1/2
  Gain2/1 -> Add1/1
  Sign1/1 -> Product4/1, 7.9+1.84=9.74/1, Product2/1, Product3/1, Product1/1, Product/1  "sign(e2(t))"
  Add1/1 -> Product/2
  Product/1 -> Add2/1  "1Pe(t)"
  Abs2/1 -> Mux/1, Variable Time Delay3/1, b11/1(In1), Variable Time Delay/1, Gain2/1  "|e2(t)|"
  Variable Time Delay/1 -> Gain5/1  "|e2(t-tau1(t))|"
  Abs3/1 -> b1/1(In1), Variable Time Delay2/1, Variable Time Delay1/1, Gain3/1  "|e1(t)|"
  Gain5/1 -> Add5/1
  Add5/1 -> Product1/2
  Product1/1 -> Add2/2  "2Q1|e(t-tau1(t))|"
  In2/1 -> Abs3/1
  b11/1(Out1) -> Add6/1
  b1/1(Out1) -> Add6/2
  Add6/1 -> Product2/2
  Product2/1 -> Add2/4  "4R Inst(t-rou(t),t))"
  Add2/1 -> Out1/1  "上面是控制器2 的各项，注意最后一项k=1,ksi=0"
  Clock1/1 -> tau2(t)=0.5(1+sin(t))/1(In1)
  tau2(t)=0.5(1+sin(t))/1(Out1) -> Variable Time Delay1/2, Variable Time Delay3/2  "tau2(t)"
  Clock/1 -> tau1(t)/1(In1)
  tau1(t)/1(Out1) -> Variable Time Delay2/2, Variable Time Delay/2  "tau1(t)"
  Product3/1 -> Add2/3  "3Q2|e(t-tau2(t))|"
  Constant/1 -> Mux/2
  Mux/1 -> Fcn/1
  Gain7/1 -> Add5/2
  Variable Time Delay2/1 -> Gain7/1
  Variable Time Delay1/1 -> Gain9/1
  Variable Time Delay3/1 -> Gain1/1
  Gain1/1 -> Add4/1
  Gain9/1 -> Add4/2
  Add4/1 -> Product3/2
  7.9+1.84=9.74/1 -> Add2/5  "5T*ksi"
  Fcn/1 -> Product4/2  "6"
  Product4/1 -> Add2/6

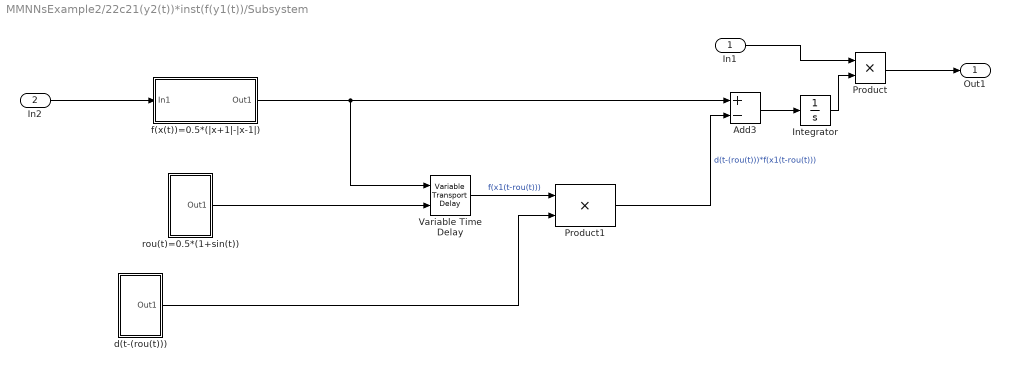
== system MMNNsExample2/22c21(y2(t))*inst(f(y1(t))/Subsystem ==
  In1 : Inport
  In2 : Inport  Port=2
  Add3 : Sum  Inputs=+-
  Integrator : Integrator  InitialCondition=0.2
      settings: AttributesFormatString=|
      | %<Name>
      | %<InitialCondition>
  Product : Product
  Product1 : Product
  Variable Time Delay : VariableTransportDelay  MaximumDelay=10  MaximumPoints=2^21
      settings: AttributesFormatString=%<Name>
  d(t-(rou(t))) : Subsystem
  f(x(t))=0.5*(|x+1|-|x-1|) : Subsystem
  rou(t)=0.5*(1+sin(t)) : Subsystem
  Out1 : Outport
  wires:
  Variable Time Delay/1 -> Product1/1  "f(x1(t-rou(t)))"
  f(x(t))=0.5*(|x+1|-|x-1|)/1(Out1) -> Variable Time Delay/1, Add3/1
  d(t-(rou(t)))/1(Out1) -> Product1/2
  Add3/1 -> Integrator/1
  rou(t)=0.5*(1+sin(t))/1(Out1) -> Variable Time Delay/2
  Product1/1 -> Add3/2  "d(t-(rou(t)))*f(x1(t-rou(t)))"
  Integrator/1 -> Product/2
  Product/1 -> Out1/1
  In1/1 -> Product/1
  In2/1 -> f(x(t))=0.5*(|x+1|-|x-1|)/1(In1)

== system MMNNsExample2/2a11(y1(t))*f(y1(t))/a11(x1(t))*x1(t) ==
  ln1 : Inport
  In2 : Inport  Port=2
      settings: AttributesFormatString=%<Name>
  Product : Product  RndMeth=Zero
  Subsystem : Subsystem
  Out1 : Outport
  wires:
  Product/1 -> Out1/1
  Subsystem/1(Out1) -> Product/1
  In2/1 -> Subsystem/1(In1)
  ln1/1 -> Product/2

== system MMNNsExample2/2a12(y1(t))*f(y2(t))/Subsystem ==
  In1 : Inport
  In2 : Inport  Port=2
  Product : Product
  f(x2(t)) : Subsystem
  Out1 : Outport
  wires:
  f(x2(t))/1(Out1) -> Product/2
  Product/1 -> Out1/1
  In2/1 -> f(x2(t))/1(In1)
  In1/1 -> Product/1

== system MMNNsExample2/2a21(y2(t))*y1(t)1/f1(x1(t))=(|x+1|-|x-1|)//2 ==
  In1 : Inport
  Abs : Abs
  Abs1 : Abs
  Add : Sum
  Add1 : Sum  Inputs=-+
  Add2 : Sum  Inputs=+-
  Constant : Constant
  Gain : Gain  Gain=0.5
  Out1 : Outport
  wires:
  Abs1/1 -> Add2/2
  Constant/1 -> Add1/1, Add/2
  Add/1 -> Abs/1
  In1/1 -> Add1/2, Add/1  "x1(t)"
  Add1/1 -> Abs1/1
  Gain/1 -> Out1/1
  Add2/1 -> Gain/1  "f=(|x+1|-|x-1|)/2"
  Abs/1 -> Add2/1

== system MMNNsExample2/2a22(x2(t))*f(x2(t))1/a22(x2(t))*x2(t) ==
  ln1 : Inport
  In2 : Inport  Port=2
  Product : Product  RndMeth=Zero
  f(x(t))=0.5*(|x+1|-|x-1|) : Subsystem
  Out1 : Outport
  wires:
  Product/1 -> Out1/1
  f(x(t))=0.5*(|x+1|-|x-1|)/1(Out1) -> Product/2
  In2/1 -> f(x(t))=0.5*(|x+1|-|x-1|)/1(In1)
  ln1/1 -> Product/1

== system MMNNsExample2/2b(1)11(y1(t))*f(y1(t-tau2(t)))/x1(t)*b11(x1(t)) ==
  In1 : Inport
  In2 : Inport  Port=2
  Product1 : Product  RndMeth=Zero
  Variable Time Delay : VariableTransportDelay  MaximumDelay=10  MaximumPoints=2^25
  f=(|x+1|-|x-1|)/2 : Subsystem
  tau2(t)=0.5+0.5*sin(t) : Subsystem
  Out1 : Outport
  wires:
  In1/1 -> Product1/1  "b11(x1(t))"
  Product1/1 -> Out1/1
  f=(|x+1|-|x-1|)/2/1(Out1) -> Variable Time Delay/1
  Variable Time Delay/1 -> Product1/2  "f1(x1(t-tau2(t)))"
  In2/1 -> f=(|x+1|-|x-1|)/2/1(In1)  "x1(t)"
  tau2(t)=0.5+0.5*sin(t)/1(tau(t)=0.5+0.5*sin(t)) -> Variable Time Delay/2

== system MMNNsExample2/2b(1)21(y2(t))*f(y1(t-tau1(t)))1/Subsystem ==
  In1 : Inport
      settings: AttributesFormatString=%<Name>
  In2 : Inport  Port=2
  Product : Product
  Variable Time Delay : VariableTransportDelay  MaximumDelay=10  MaximumPoints=2^25
      settings: AttributesFormatString=%<Name>
  f(x(t))=0.5*(|x+1|-|x-1|) : Subsystem
  tau(t)=0.5+0.5*cos(t) : Subsystem
  Out1 : Outport
      settings: AttributesFormatString=%<Name>
  wires:
  Variable Time Delay/1 -> Product/2  "f(x1(t-tau(t))"
  f(x(t))=0.5*(|x+1|-|x-1|)/1(Out1) -> Variable Time Delay/1
  tau(t)=0.5+0.5*cos(t)/1(Out1) -> Variable Time Delay/2
  Product/1 -> Out1/1
  In1/1 -> Product/1
  In2/1 -> f(x(t))=0.5*(|x+1|-|x-1|)/1(In1)

== system MMNNsExample2/2b(1)22(y2(t))*f(y2(t-tau(t))1/x2(t)*b22(x2(t)) ==
  In1 : Inport
  In2 : Inport  Port=2
  Product1 : Product  RndMeth=Zero
  Variable Time Delay : VariableTransportDelay  MaximumDelay=10  MaximumPoints=2^25
  f(x(t))=0.5*(|x+1|-|x-1|) : Subsystem
  tau(t)=0.5+0.5*cos(t) : Subsystem
  Out1 : Outport
  wires:
  Product1/1 -> Out1/1
  f(x(t))=0.5*(|x+1|-|x-1|)/1(Out1) -> Variable Time Delay/1
  Variable Time Delay/1 -> Product1/2  "f2(x2(t-tau(t)))"
  tau(t)=0.5+0.5*cos(t)/1(Out1) -> Variable Time Delay/2
  In2/1 -> f(x(t))=0.5*(|x+1|-|x-1|)/1(In1)  "x2(t)"
  In1/1 -> Product1/1  "b22(x2(t))"

== system MMNNsExample2/2b(2)12(y1(t))*f(y2(t-tau2(t)))/Subsystem ==
  In1 : Inport
      settings: AttributesFormatString=%<Name>
  In2 : Inport  Port=2
      settings: AttributesFormatString=%<Name>
  Product : Product
  Variable Time Delay : VariableTransportDelay  MaximumDelay=10  MaximumPoints=2^25
      settings: AttributesFormatString=%<Name>
  f=(|x+1|-|x-1|)/2 : Subsystem
  tau(t)=0.5+0.5*sin(t) : Subsystem
  Out1 : Outport
  wires:
  tau(t)=0.5+0.5*sin(t)/1(Out1) -> Variable Time Delay/2
  In1/1 -> Product/1
  Variable Time Delay/1 -> Product/2  "f(x2(t-tau2(t))"
  f=(|x+1|-|x-1|)/2/1(Out1) -> Variable Time Delay/1
  Product/1 -> Out1/1
  In2/1 -> f=(|x+1|-|x-1|)/2/1(In1)

== system MMNNsExample2/2b(2)21(y2(t))*f(y1(t-tau2(t)))1/Subsystem ==
  In1 : Inport
      settings: AttributesFormatString=%<Name>
  In2 : Inport  Port=2
  Product : Product
  Variable Time Delay : VariableTransportDelay  MaximumDelay=10  MaximumPoints=2^25
      settings: AttributesFormatString=%<Name>
  f(x(t))=0.5*(|x+1|-|x-1|) : Subsystem
  tau(t)=0.5+0.5*sin(t) : Subsystem
  Out1 : Outport
      settings: AttributesFormatString=%<Name>
  wires:
  Variable Time Delay/1 -> Product/2  "f(x1(t-tau(t))"
  f(x(t))=0.5*(|x+1|-|x-1|)/1(Out1) -> Variable Time Delay/1
  tau(t)=0.5+0.5*sin(t)/1(Out1) -> Variable Time Delay/2
  Product/1 -> Out1/1
  In1/1 -> Product/1
  In2/1 -> f(x(t))=0.5*(|x+1|-|x-1|)/1(In1)

== system MMNNsExample2/2b(2)22(y2(t))*f(y2(t-tau2(t))/x2(t)*b22(x2(t)) ==
  In1 : Inport
  In2 : Inport  Port=2
  Product1 : Product  RndMeth=Zero
  Variable Time Delay : VariableTransportDelay  MaximumDelay=10  MaximumPoints=2^25
  f(x(t))=0.5*(|x+1|-|x-1|) : Subsystem
  tau(t)=0.5+0.5*sin(t) : Subsystem
  Out1 : Outport
  wires:
  Product1/1 -> Out1/1
  f(x(t))=0.5*(|x+1|-|x-1|)/1(Out1) -> Variable Time Delay/1
  Variable Time Delay/1 -> Product1/2  "f2(x2(t-tau2(t)))"
  tau(t)=0.5+0.5*sin(t)/1(Out1) -> Variable Time Delay/2
  In2/1 -> f(x(t))=0.5*(|x+1|-|x-1|)/1(In1)  "x2(t)"
  In1/1 -> Product1/1  "b22(x2(t))"

== system MMNNsExample2/2b11(y1(t))*f(y1(t-tau(t)))/x1(t)*b11(x1(t)) ==
  In1 : Inport
  In2 : Inport  Port=2
  Product1 : Product  RndMeth=Zero
  Variable Time Delay : VariableTransportDelay  MaximumDelay=10  MaximumPoints=2^25
  f=(|x+1|-|x-1|)/2 : Subsystem
  tau(t)=0.5+0.5*cos(t) : Subsystem
  Out1 : Outport
  wires:
  In1/1 -> Product1/1  "b11(x1(t))"
  Product1/1 -> Out1/1
  f=(|x+1|-|x-1|)/2/1(Out1) -> Variable Time Delay/1
  Variable Time Delay/1 -> Product1/2  "f1(x1(t-tau(t)))"
  In2/1 -> f=(|x+1|-|x-1|)/2/1(In1)  "x1(t)"
  tau(t)=0.5+0.5*cos(t)/1(tau(t)=0.5+0.5*cos(t)) -> Variable Time Delay/2

== system MMNNsExample2/2b12(y1(t))*f(y2(t-tau1(t)))/Subsystem ==
  In1 : Inport
      settings: AttributesFormatString=%<Name>
  In2 : Inport  Port=2
      settings: AttributesFormatString=%<Name>
  Product : Product
  Variable Time Delay : VariableTransportDelay  MaximumDelay=10  MaximumPoints=2^25
      settings: AttributesFormatString=%<Name>
  f=(|x+1|-|x-1|)/2 : Subsystem
  tau(t)=0.5+0.5*cos(t) : Subsystem
  Out1 : Outport
  wires:
  tau(t)=0.5+0.5*cos(t)/1(Out1) -> Variable Time Delay/2
  In1/1 -> Product/1
  Variable Time Delay/1 -> Product/2  "f(x2(t-tau(t))"
  f=(|x+1|-|x-1|)/2/1(Out1) -> Variable Time Delay/1
  Product/1 -> Out1/1
  In2/1 -> f=(|x+1|-|x-1|)/2/1(In1)

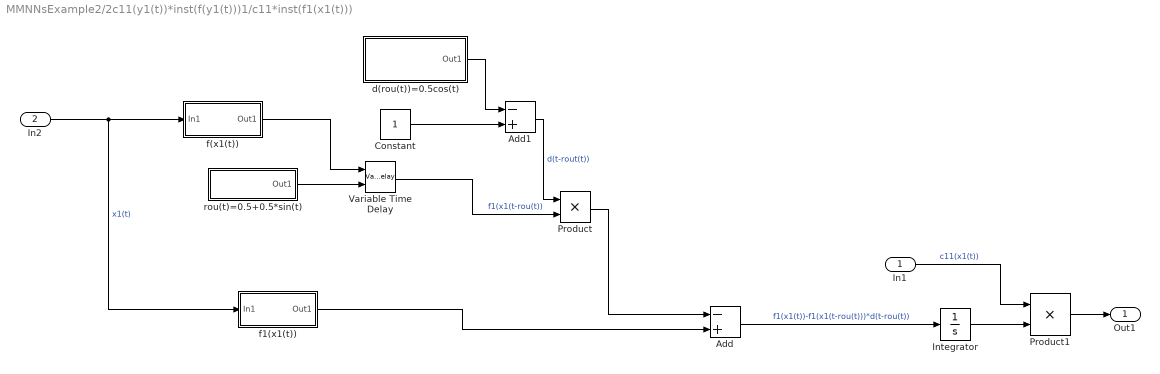
== system MMNNsExample2/2c11(y1(t))*inst(f(y1(t)))1/c11*inst(f1(x1(t))) ==
  In1 : Inport
  In2 : Inport  Port=2
  Add : Sum  Inputs=-+
  Add1 : Sum  Inputs=-+
  Constant : Constant
  Integrator : Integrator  InitialCondition=0.2
      settings: AttributesFormatString=|
      | %<Name>
      | %<InitialCondition>
  Product : Product
  Product1 : Product  RndMeth=Zero
  Variable Time Delay : VariableTransportDelay  MaximumDelay=10  MaximumPoints=2^21
  d(rou(t))=0.5cos(t) : Subsystem
  f(x1(t)) : Subsystem
  f1(x1(t)) : Subsystem
  rou(t)=0.5+0.5*sin(t) : Subsystem
  Out1 : Outport
  wires:
  Product1/1 -> Out1/1
  f(x1(t))/1(Out1) -> Variable Time Delay/1
  rou(t)=0.5+0.5*sin(t)/1(Out1) -> Variable Time Delay/2
  f1(x1(t))/1(Out1) -> Add/2
  Constant/1 -> Add1/2
  d(rou(t))=0.5cos(t)/1(Out1) -> Add1/1
  Add1/1 -> Product/1  "d(t-rout(t))"
  Variable Time Delay/1 -> Product/2  "f1(x1(t-rou(t))"
  Product/1 -> Add/1
  Add/1 -> Integrator/1  "f1(x1(t))-f1(x1(t-rou(t)))*d(t-rou(t))"
  Integrator/1 -> Product1/2
  In2/1 -> f1(x1(t))/1(In1), f(x1(t))/1(In1)  "x1(t)"
  In1/1 -> Product1/1  "c11(x1(t))"

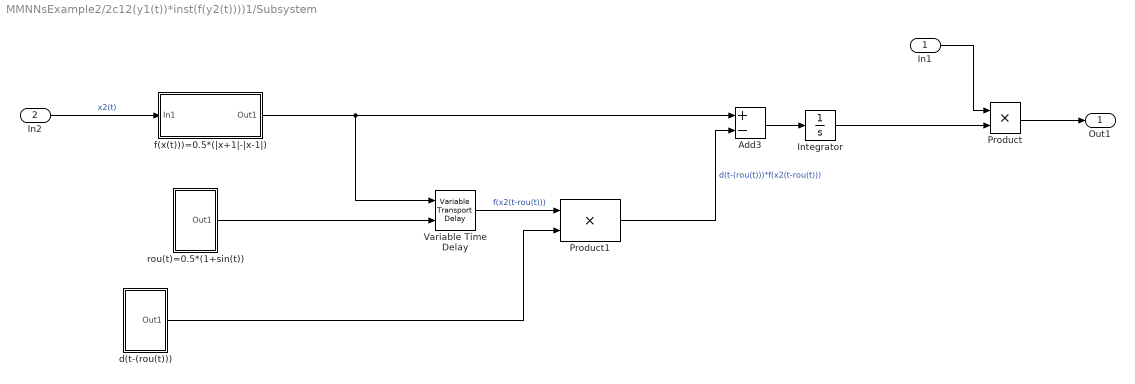
== system MMNNsExample2/2c12(y1(t))*inst(f(y2(t))))1/Subsystem ==
  In1 : Inport
      settings: AttributesFormatString=%<Name>
  In2 : Inport  Port=2
      settings: AttributesFormatString=%<Name>
  Add3 : Sum  Inputs=+-
  Integrator : Integrator  InitialCondition=0.3
      settings: AttributesFormatString=|
      | %<Name>
      | %<InitialCondition>
  Product : Product
  Product1 : Product
  Variable Time Delay : VariableTransportDelay  MaximumDelay=10  MaximumPoints=2^21
      settings: AttributesFormatString=%<Name>
  d(t-(rou(t))) : Subsystem
  f(x(t)))=0.5*(|x+1|-|x-1|) : Subsystem
  rou(t)=0.5*(1+sin(t)) : Subsystem
  Out1 : Outport
      settings: AttributesFormatString=%<Name>
  wires:
  f(x(t)))=0.5*(|x+1|-|x-1|)/1(Out1) -> Variable Time Delay/1, Add3/1
  Add3/1 -> Integrator/1
  d(t-(rou(t)))/1(Out1) -> Product1/2
  rou(t)=0.5*(1+sin(t))/1(Out1) -> Variable Time Delay/2
  Variable Time Delay/1 -> Product1/1  "f(x2(t-rou(t)))"
  Product1/1 -> Add3/2  "d(t-(rou(t)))*f(x2(t-rou(t)))"
  Integrator/1 -> Product/2
  In1/1 -> Product/1
  In2/1 -> f(x(t)))=0.5*(|x+1|-|x-1|)/1(In1)  "x2(t)"
  Product/1 -> Out1/1

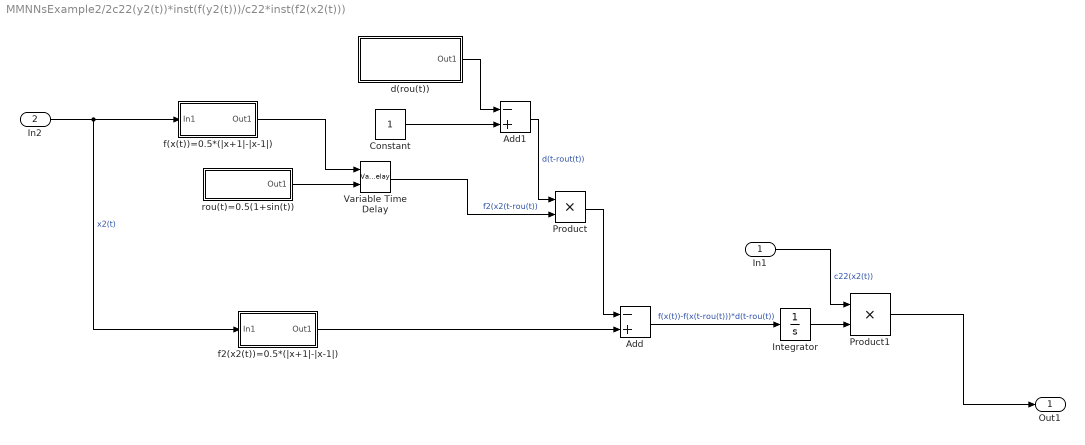
== system MMNNsExample2/2c22(y2(t))*inst(f(y2(t)))/c22*inst(f2(x2(t))) ==
  In1 : Inport
  In2 : Inport  Port=2
  Add : Sum  Inputs=-+
  Add1 : Sum  Inputs=-+
  Constant : Constant
  Integrator : Integrator  InitialCondition=0.3
      settings: AttributesFormatString=|
      | %<Name>
      | %<InitialCondition>
  Product : Product
  Product1 : Product  RndMeth=Zero
  Variable Time Delay : VariableTransportDelay  MaximumDelay=10  MaximumPoints=2^21
  d(rou(t)) : Subsystem
  f(x(t))=0.5*(|x+1|-|x-1|) : Subsystem
  f2(x2(t))=0.5*(|x+1|-|x-1|) : Subsystem
  rou(t)=0.5(1+sin(t)) : Subsystem
  Out1 : Outport
  wires:
  Product1/1 -> Out1/1
  f(x(t))=0.5*(|x+1|-|x-1|)/1(Out1) -> Variable Time Delay/1
  rou(t)=0.5(1+sin(t))/1(Out1) -> Variable Time Delay/2
  f2(x2(t))=0.5*(|x+1|-|x-1|)/1(Out1) -> Add/2
  Constant/1 -> Add1/2
  d(rou(t))/1(Out1) -> Add1/1
  Add1/1 -> Product/1  "d(t-rout(t))"
  Variable Time Delay/1 -> Product/2  "f2(x2(t-rou(t))"
  Product/1 -> Add/1
  Add/1 -> Integrator/1  "f(x(t))-f(x(t-rou(t)))*d(t-rou(t))"
  Integrator/1 -> Product1/2
  In2/1 -> f2(x2(t))=0.5*(|x+1|-|x-1|)/1(In1), f(x(t))=0.5*(|x+1|-|x-1|)/1(In1)  "x2(t)"
  In1/1 -> Product1/1  "c22(x2(t))"

== system MMNNsExample2/a11(x1(t))*f(x1(t))/a11(x1(t))*x1(t) ==
  ln1 : Inport
  In2 : Inport  Port=2
      settings: AttributesFormatString=%<Name>
  Product : Product  RndMeth=Zero
  Subsystem : Subsystem
  Out1 : Outport
  wires:
  Product/1 -> Out1/1
  Subsystem/1(Out1) -> Product/1
  In2/1 -> Subsystem/1(In1)
  ln1/1 -> Product/2

== system MMNNsExample2/a12(x1(t))*f(x2(t))/Subsystem ==
  In1 : Inport
  In2 : Inport  Port=2
  Product : Product
  f(x2(t)) : Subsystem
  Out1 : Outport
  wires:
  f(x2(t))/1(Out1) -> Product/2
  Product/1 -> Out1/1
  In2/1 -> f(x2(t))/1(In1)
  In1/1 -> Product/1

== system MMNNsExample2/a21(x2(t))*f(x1(t))/f1(x1(t))=(|x+1|-|x-1|)//2 ==
  In1 : Inport
  Abs : Abs
  Abs1 : Abs
  Add : Sum
  Add1 : Sum  Inputs=-+
  Add2 : Sum  Inputs=+-
  Constant : Constant
  Gain : Gain  Gain=0.5
  Out1 : Outport
  wires:
  Abs1/1 -> Add2/2
  Constant/1 -> Add1/1, Add/2
  Add/1 -> Abs/1
  In1/1 -> Add1/2, Add/1  "x1(t)"
  Add1/1 -> Abs1/1
  Gain/1 -> Out1/1
  Add2/1 -> Gain/1  "f=(|x+1|-|x-1|)/2"
  Abs/1 -> Add2/1

== system MMNNsExample2/a22(x2(t))*f(x2(t))/a22(x2(t))*x2(t) ==
  ln1 : Inport
  In2 : Inport  Port=2
  Product : Product  RndMeth=Zero
  f(x(t))=0.5*(|x+1|-|x-1|) : Subsystem
  Out1 : Outport
  wires:
  Product/1 -> Out1/1
  f(x(t))=0.5*(|x+1|-|x-1|)/1(Out1) -> Product/2
  In2/1 -> f(x(t))=0.5*(|x+1|-|x-1|)/1(In1)
  ln1/1 -> Product/1

== system MMNNsExample2/b(1)12(x1(t))*f(x2(t-tau1(t)))/Subsystem ==
  In1 : Inport
      settings: AttributesFormatString=%<Name>
  In2 : Inport  Port=2
      settings: AttributesFormatString=%<Name>
  Product : Product
  Variable Time Delay : VariableTransportDelay  MaximumDelay=10  MaximumPoints=2^25
      settings: AttributesFormatString=%<Name>
  f=(|x+1|-|x-1|)/2 : Subsystem
  tau(t)=0.5+0.5*cos(t) : Subsystem
  Out1 : Outport
  wires:
  tau(t)=0.5+0.5*cos(t)/1(Out1) -> Variable Time Delay/2
  In1/1 -> Product/1
  Variable Time Delay/1 -> Product/2  "f(x2(t-tau(t))"
  f=(|x+1|-|x-1|)/2/1(Out1) -> Variable Time Delay/1
  Product/1 -> Out1/1
  In2/1 -> f=(|x+1|-|x-1|)/2/1(In1)

== system MMNNsExample2/b(1)21(x2(t))*f(x1(t-tau1(t)))/Subsystem ==
  In1 : Inport
      settings: AttributesFormatString=%<Name>
  In2 : Inport  Port=2
  Product : Product
  Variable Time Delay : VariableTransportDelay  MaximumDelay=10  MaximumPoints=2^21
      settings: AttributesFormatString=%<Name>
  f(x(t))=0.5*(|x+1|-|x-1|) : Subsystem
  tau(t)=0.5+0.5*cos(t) : Subsystem
  Out1 : Outport
      settings: AttributesFormatString=%<Name>
  wires:
  Variable Time Delay/1 -> Product/2  "f(x1(t-tau(t))"
  f(x(t))=0.5*(|x+1|-|x-1|)/1(Out1) -> Variable Time Delay/1
  tau(t)=0.5+0.5*cos(t)/1(Out1) -> Variable Time Delay/2
  Product/1 -> Out1/1
  In1/1 -> Product/1
  In2/1 -> f(x(t))=0.5*(|x+1|-|x-1|)/1(In1)  "x1(t)"
